simulink library "reaction_wheel_assembly_lib"  (R2018b)
settings: Solver=VariableStepAuto  StartTime=0.0  StopTime=10.0  RelTol=1e-3
undefined symbols (not defined in the file or in its folder): sim_params
libraries: reaction_wheel_PID_lib x4, rw_motor_lib x4, rw_valid_lib x1
settings Model: Creator=unsik  LastModifiedBy=Taylor
settings SFSimCC: SimUseLocalCustomCode=off
settings RTWCC: RTWUseLocalCustomCode=off
settings CodeAppCC: StateflowObjectComments=on

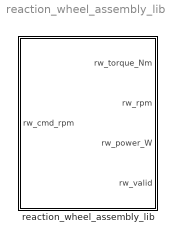
== system reaction_wheel_assembly_lib ==
  reaction_wheel_assembly_lib : Subsystem

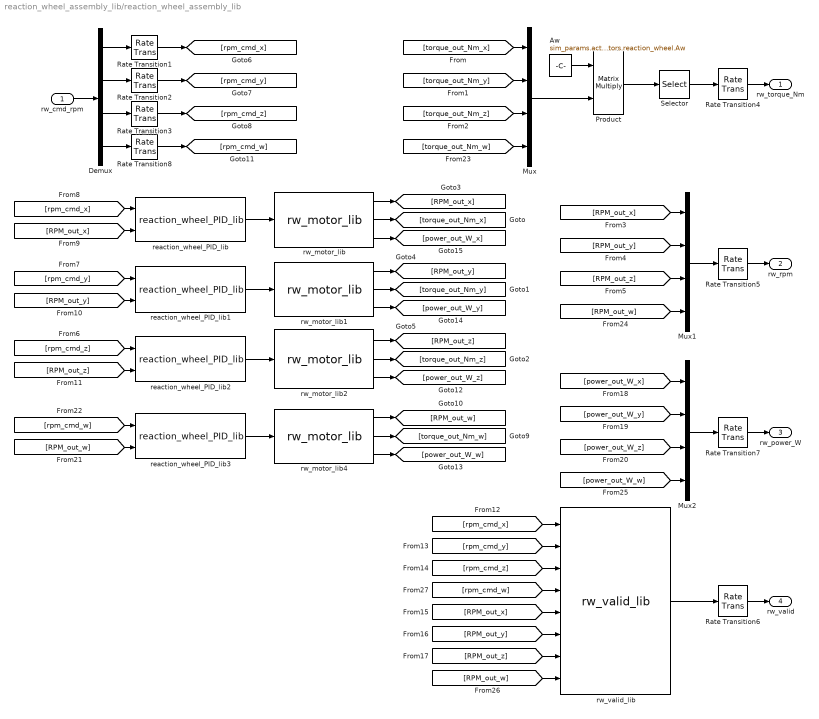
== system reaction_wheel_assembly_lib/reaction_wheel_assembly_lib ==
  rw_cmd_rpm : Inport
  Aw : Constant  Value=sim_params.actuators.reaction_wheel.Aw
  Demux : Demux
  Mux : Mux
  Mux1 : Mux
  Mux2 : Mux
  Product : Product  Multiplication=Matrix(*)
  Rate Transition{1..3,8} (4 alike) : RateTransition  InitialCondition=sim_params.actuators.reaction_wheel.ic.rt1  OutPortSampleTime=sim_params.actuators.reaction_wheel.sample_time_s
  Rate Transition4 : RateTransition
  Rate Transition5 : RateTransition  InitialCondition=sim_params.actuators.reaction_wheel.ic.rpm
  Rate Transition6 : RateTransition
  Rate Transition7 : RateTransition  InitialCondition=sim_params.actuators.reaction_wheel.ic.rpm
  Selector : Selector  InputPortWidth=4  IndexOptions=Index vector (dialog)  Indices=[1 2 3]  OutputSizes=1
  reaction_wheel_PID_lib{,1..3} (4 alike) : reaction_wheel_PID_lib/reaction_wheel_PID_lib  SystemSampleTime=-1
  rw_motor_lib{,1..2,4} (4 alike) : rw_motor_lib/rw_motor_lib  SystemSampleTime=-1
  rw_valid_lib : rw_valid_lib/rw_valid_lib  SystemSampleTime=-1
  rw_torque_Nm : Outport
  rw_rpm : Outport  Port=2
  rw_power_W : Outport  Port=3
  rw_valid : Outport  Port=4
  wires:
  [power_out_W_w] -> Mux2/4
  [power_out_W_z] -> Mux2/3
  [power_out_W_y] -> Mux2/2
  [power_out_W_x] -> Mux2/1
  [RPM_out_w] -> Mux1/4
  [torque_out_Nm_w] -> Mux/4
  rw_motor_lib/3 -> [power_out_W_x]
  rw_motor_lib1/3 -> [power_out_W_y]
  Rate Transition8/1 -> [rpm_cmd_w]
  Demux/4 -> Rate Transition8/1
  rw_motor_lib4/3 -> [power_out_W_w]
  [RPM_out_w] -> reaction_wheel_PID_lib3/2
  reaction_wheel_PID_lib3/1 -> rw_motor_lib4/1
  rw_motor_lib4/1 -> [RPM_out_w]
  [rpm_cmd_w] -> reaction_wheel_PID_lib3/1
  rw_motor_lib4/2 -> [torque_out_Nm_w]
  Mux2/1 -> Rate Transition7/1
  Rate Transition7/1 -> rw_power_W/1
  rw_motor_lib2/3 -> [power_out_W_z]
  reaction_wheel_PID_lib/1 -> rw_motor_lib/1
  Rate Transition1/1 -> [rpm_cmd_x]
  reaction_wheel_PID_lib1/1 -> rw_motor_lib1/1
  reaction_wheel_PID_lib2/1 -> rw_motor_lib2/1
  Demux/1 -> Rate Transition1/1
  Demux/2 -> Rate Transition2/1
  Demux/3 -> Rate Transition3/1
  rw_cmd_rpm/1 -> Demux/1
  [torque_out_Nm_x] -> Mux/1
  [torque_out_Nm_y] -> Mux/2
  [torque_out_Nm_z] -> Mux/3
  rw_motor_lib1/2 -> [torque_out_Nm_y]
  rw_motor_lib2/2 -> [torque_out_Nm_z]
  [RPM_out_x] -> Mux1/1
  [RPM_out_y] -> Mux1/2
  [RPM_out_z] -> Mux1/3
  rw_motor_lib/2 -> [torque_out_Nm_x]
  rw_motor_lib/1 -> [RPM_out_x]
  rw_motor_lib2/1 -> [RPM_out_z]
  rw_motor_lib1/1 -> [RPM_out_y]
  [RPM_out_x] -> reaction_wheel_PID_lib/2
  [RPM_out_y] -> reaction_wheel_PID_lib1/2
  [RPM_out_z] -> reaction_wheel_PID_lib2/2
  Rate Transition4/1 -> rw_torque_Nm/1
  Mux1/1 -> Rate Transition5/1
  Rate Transition5/1 -> rw_rpm/1
  Rate Transition3/1 -> [rpm_cmd_z]
  Rate Transition2/1 -> [rpm_cmd_y]
  [rpm_cmd_z] -> reaction_wheel_PID_lib2/1
  [rpm_cmd_y] -> reaction_wheel_PID_lib1/1
  [rpm_cmd_x] -> reaction_wheel_PID_lib/1
  [rpm_cmd_x] -> rw_valid_lib/1
  [rpm_cmd_y] -> rw_valid_lib/2
  [rpm_cmd_z] -> rw_valid_lib/3
  rw_valid_lib/1 -> Rate Transition6/1
  Rate Transition6/1 -> rw_valid/1
  Mux/1 -> Product/2
  Aw/1 -> Product/1
  Product/1 -> Selector/1
  Selector/1 -> Rate Transition4/1
  [rpm_cmd_w] -> rw_valid_lib/4
  [RPM_out_z] -> rw_valid_lib/7
  [RPM_out_x] -> rw_valid_lib/5
  [RPM_out_y] -> rw_valid_lib/6
  [RPM_out_w] -> rw_valid_lib/8
